simulink model "Concave_hipp"  (R2023a)
settings: Solver=ode3  StartTime=0.0  StopTime=100  FixedStep=0.0001  RelTol=1e-3
values from neighbouring files (symbols this model uses):
  d_pitch_2 = 1    [simulation_para.m]
  d_roll_2 = 1    [simulation_para.m]
  d_yaw_2 = 1    [simulation_para.m]
  disturbance = 0    [simulation_para.m]
  dpitch_para = [1,1,1,0.01]    [simulation_para.m]
  droll_para = [1,1,1,0.01]    [simulation_para.m]
  dyaw_para = [1,1,1,0.01]    [simulation_para.m]
  k_pos_2 = 8    [simulation_para.m]
  k_vel_2 = 8    [simulation_para.m]
  kp_para = [8,20,1,0.01]    [simulation_para.m]
  kv_para = [8,20,1,0.01]    [simulation_para.m]
  p_pitch_2 = 10    [simulation_para.m]
  p_roll_2 = 10    [simulation_para.m]
  p_yaw_2 = 10    [simulation_para.m]
  ppitch_para = [10,10,1,0.01]    [simulation_para.m]
  proll_para = [10,10,1,0.01]    [simulation_para.m]
  pyaw_para = [10,20,1,0.01]    [simulation_para.m]
  Q1 = -8    [simulation_para.m]
  Q2 = -10    [simulation_para.m]
  Q3 = -[0.01,5,8]    [simulation_para.m]
  Q4 = -[0.001,0.1,0.1]    [simulation_para.m]
  Qc1 = -[8,50,1,0.01]    [simulation_para.m]
  Qc2 = -[10,80,1,0.02]    [simulation_para.m]
  Qc3 = [qc3_1;qc3_2;qc3_3]    [simulation_para.m]
  Qc4 = [qc4_1;qc4_2;qc4_3]    [simulation_para.m]
(part 1 of 2)
settings Model: Creator=fansh  LastModifiedBy=fansh
settings DebuggingCC: MultiTaskCondExecSysMsg=none  MultiTaskRateTransMsg=warning  TasksWithSamePriorityMsg=none  SigSpecEnsureSampleTimeMsg=none  UnknownTsInhSupMsg=none  SFUnexpectedBacktrackingDiag=none

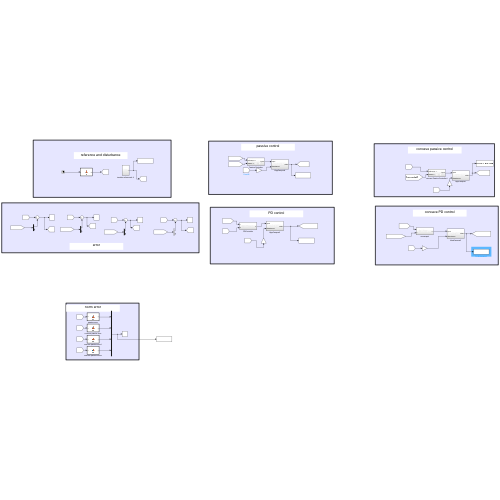
[thumbnail: Simulink's stored preview of the top-level diagram]
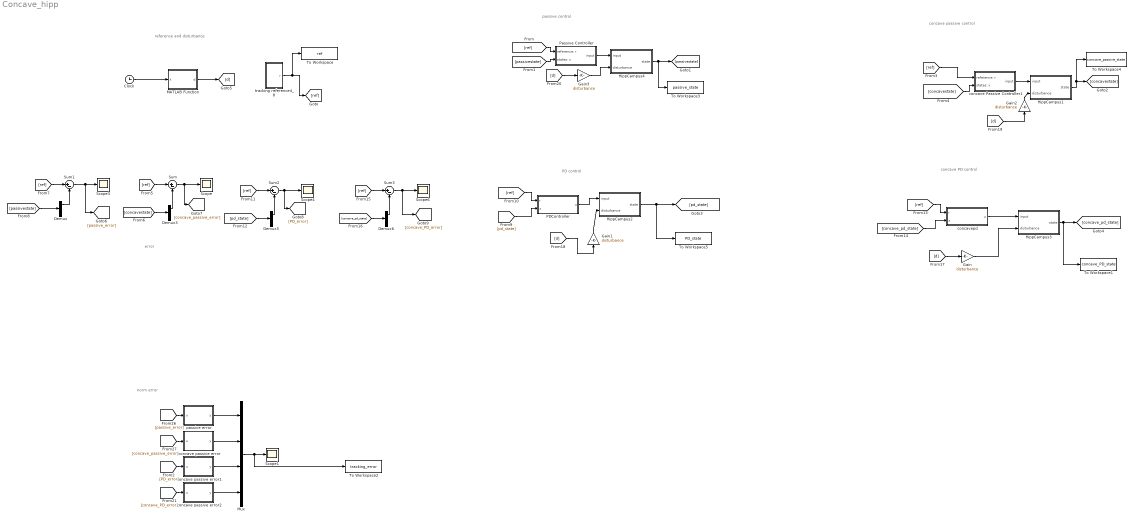
== system Concave_hipp ==
  note: concave passive control
  note: passive control
  note: PD control
  note: concave PD control
  note: reference and disturbance
  note: error
  note: norm error
  Clock : Clock
  Demux{,3,5..6} (4 alike) : Demux  Outputs=[3 9]
  Gain{,1..3} (4 alike) : Gain  Gain=disturbance
  HippCampus1 : Subsystem
  HippCampus2 : Subsystem
  HippCampus3 : Subsystem
  HippCampus4 : Subsystem
  MATLAB Function : MATLAB Function  TreatAsAtomicUnit=on
  Mux : Mux
  PDController : Subsystem
  Passive Controller : Subsystem
  Scope{,1,3..4,6} (5 alike) : Scope
  Sum{,1..3} (4 alike) : Sum  Inputs=|+-
  To Workspace : ToWorkspace  VariableName=ref  SaveFormat=Timeseries  SampleTime=-1
  To Workspace1 : ToWorkspace  VariableName=concave_PD_state  SaveFormat=Timeseries  SampleTime=-1
  To Workspace2 : ToWorkspace  VariableName=tracking_error  SaveFormat=Timeseries  SampleTime=-1
  To Workspace3 : ToWorkspace  VariableName=passive_state  SaveFormat=Timeseries  SampleTime=-1
  To Workspace4 : ToWorkspace  VariableName=concave_passive_state  SaveFormat=Timeseries  SampleTime=-1
  To Workspace5 : ToWorkspace  VariableName=PD_state  SaveFormat=Timeseries  SampleTime=-1
  concave Passive Controller1 : Subsystem
  concave passive error : MATLAB Function  TreatAsAtomicUnit=on
  concave passive error1 : MATLAB Function  TreatAsAtomicUnit=on
  concave passive error2 : MATLAB Function  TreatAsAtomicUnit=on
  concavepd : Subsystem
  passive error : MATLAB Function  TreatAsAtomicUnit=on
  tracking reference4_8 : Subsystem
  wires:
  Passive Controller/1(input) -> HippCampus4/1(input)
  HippCampus4/1(state) -> To Workspace3/1, [passivestate]
  [ref] -> Passive Controller/1(reference: r)
  [passivestate] -> Passive Controller/2(states: x)
  [ref] -> concave Passive Controller1/1(reference: r)
  concave Passive Controller1/1(input) -> HippCampus1/1(input)
  [concavestate] -> concave Passive Controller1/2(states: x)
  HippCampus1/1(state) -> To Workspace4/1, [concavestate]
  [ref] -> Sum/1
  [concavestate] -> Demux3/1
  Sum/1 -> [concave_passive_error], Scope/1
  [passivestate] -> Demux/1
  Sum1/1 -> [passive_error], Scope3/1
  [ref] -> Sum1/1
  Demux/1 -> Sum1/2
  Demux3/1 -> Sum/2
  PDController/1(u) -> HippCampus2/1(input)
  [ref] -> PDController/1(r)
  HippCampus2/1(state) -> To Workspace5/1, [pd_state]
  [pd_state] -> PDController/2(x)
  Sum2/1 -> [PD_error], Scope4/1
  [ref] -> Sum2/1
  [pd_state] -> Demux5/1
  Demux5/1 -> Sum2/2
  [ref] -> concavepd/1(r)
  HippCampus3/1(state) -> To Workspace1/1, [concave_pd_state]
  [concave_pd_state] -> concavepd/2(x)
  concavepd/1(u) -> HippCampus3/1(input)
  [concave_pd_state] -> Demux6/1
  [ref] -> Sum3/1
  Demux6/1 -> Sum3/2
  Sum3/1 -> [concave_PD_error], Scope6/1
  Clock/1 -> MATLAB Function/1(t)
  MATLAB Function/1(d) -> [d]
  [d] -> Gain/1
  tracking reference4_8/1(r) -> [ref], To Workspace/1
  Gain/1 -> HippCampus3/2(disturbance)
  [d] -> Gain1/1
  [d] -> Gain2/1
  [d] -> Gain3/1
  Gain1/1 -> HippCampus2/2(disturbance)
  Gain2/1 -> HippCampus1/2(disturbance)
  Gain3/1 -> HippCampus4/2(disturbance)
  [passive_error] -> passive error/1(u)
  [concave_passive_error] -> concave passive error/1(u)
  [PD_error] -> concave passive error1/1(u)
  [concave_PD_error] -> concave passive error2/1(u)
  passive error/1(y) -> Mux/1
  concave passive error/1(y) -> Mux/2
  concave passive error1/1(y) -> Mux/3
  concave passive error2/1(y) -> Mux/4
  Mux/1 -> To Workspace2/1, Scope1/1

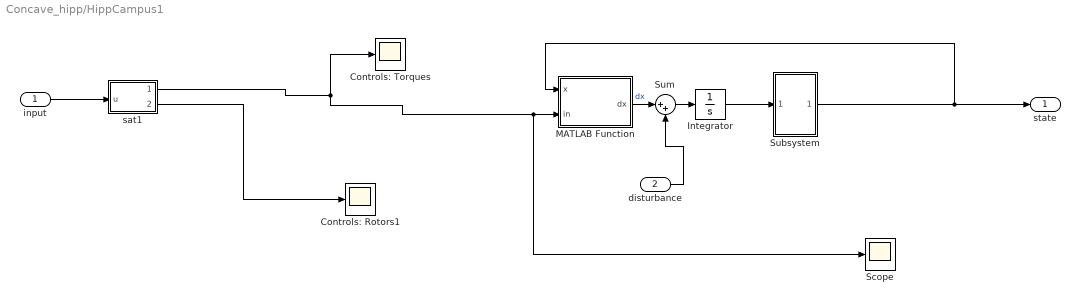
== system Concave_hipp/HippCampus1 ==
  input : Inport
  disturbance : Inport  Port=2
  Controls: Rotors1 : Scope
  Controls: Torques : Scope
  Integrator : Integrator  InitialCondition=zeros(12,1)
  MATLAB Function : MATLAB Function  TreatAsAtomicUnit=on
  Scope : Scope
  Subsystem : Subsystem
  Sum : Sum  Inputs=|++
  sat1 : MATLAB Function  TreatAsAtomicUnit=on
  state : Outport
  wires:
  MATLAB Function/1(dx) -> Sum/1  "dx"
  Integrator/1 -> Subsystem/1(In1)
  sat1/1(u_sat) -> Controls: Torques/1, MATLAB Function/2(in), Scope/1
  Subsystem/1(state) -> MATLAB Function/1(x), state/1
  input/1 -> sat1/1(u)
  sat1/2(omega) -> Controls: Rotors1/1
  Sum/1 -> Integrator/1
  disturbance/1 -> Sum/2

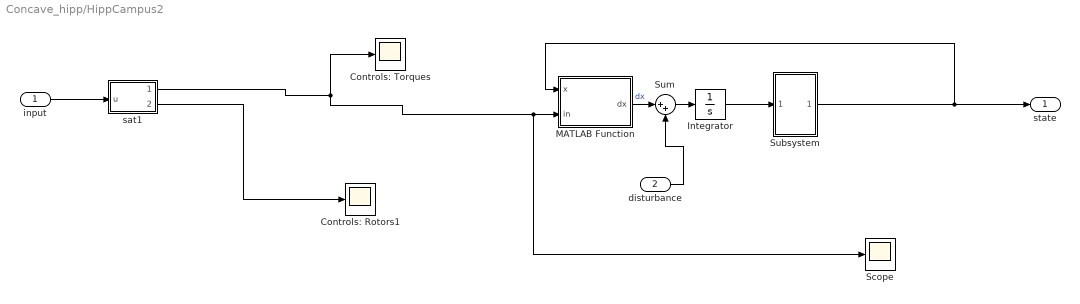
== system Concave_hipp/HippCampus2 ==
  input : Inport
  disturbance : Inport  Port=2
  Controls: Rotors1 : Scope
  Controls: Torques : Scope
  Integrator : Integrator  InitialCondition=zeros(12,1)
  MATLAB Function : MATLAB Function  TreatAsAtomicUnit=on
  Scope : Scope
  Subsystem : Subsystem
  Sum : Sum  Inputs=|++
  sat1 : MATLAB Function  TreatAsAtomicUnit=on
  state : Outport
  wires:
  MATLAB Function/1(dx) -> Sum/1  "dx"
  Integrator/1 -> Subsystem/1(In1)
  sat1/1(u_sat) -> Controls: Torques/1, MATLAB Function/2(in), Scope/1
  Subsystem/1(state) -> MATLAB Function/1(x), state/1
  input/1 -> sat1/1(u)
  sat1/2(omega) -> Controls: Rotors1/1
  Sum/1 -> Integrator/1
  disturbance/1 -> Sum/2

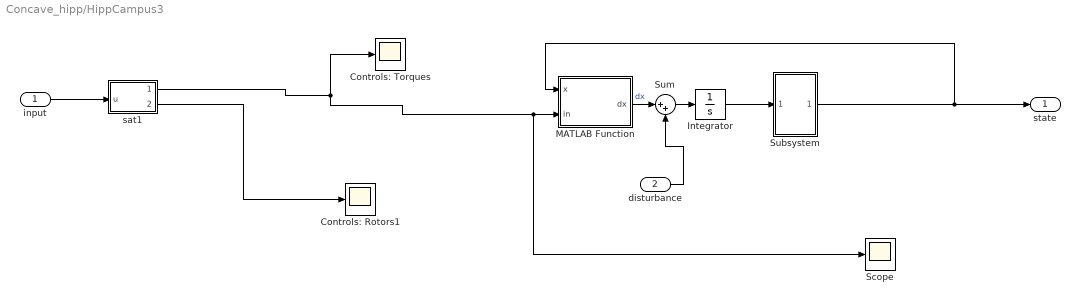
== system Concave_hipp/HippCampus3 ==
  input : Inport
  disturbance : Inport  Port=2
  Controls: Rotors1 : Scope
  Controls: Torques : Scope
  Integrator : Integrator  InitialCondition=zeros(12,1)
  MATLAB Function : MATLAB Function  TreatAsAtomicUnit=on
  Scope : Scope
  Subsystem : Subsystem
  Sum : Sum  Inputs=|++
  sat1 : MATLAB Function  TreatAsAtomicUnit=on
  state : Outport
  wires:
  MATLAB Function/1(dx) -> Sum/1  "dx"
  Integrator/1 -> Subsystem/1(In1)
  sat1/1(u_sat) -> Controls: Torques/1, MATLAB Function/2(in), Scope/1
  Subsystem/1(state) -> MATLAB Function/1(x), state/1
  input/1 -> sat1/1(u)
  sat1/2(omega) -> Controls: Rotors1/1
  Sum/1 -> Integrator/1
  disturbance/1 -> Sum/2

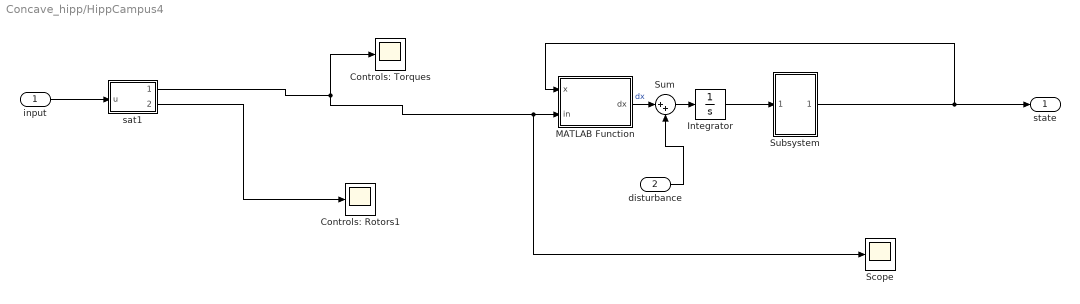
== system Concave_hipp/HippCampus4 ==
  input : Inport
  disturbance : Inport  Port=2
  Controls: Rotors1 : Scope
  Controls: Torques : Scope
  Integrator : Integrator  InitialCondition=zeros(12,1)
  MATLAB Function : MATLAB Function  TreatAsAtomicUnit=on
  Scope : Scope
  Subsystem : Subsystem
  Sum : Sum  Inputs=|++
  sat1 : MATLAB Function  TreatAsAtomicUnit=on
  state : Outport
  wires:
  MATLAB Function/1(dx) -> Sum/1  "dx"
  Integrator/1 -> Subsystem/1(In1)
  sat1/1(u_sat) -> Controls: Torques/1, MATLAB Function/2(in), Scope/1
  Subsystem/1(state) -> MATLAB Function/1(x), state/1
  input/1 -> sat1/1(u)
  sat1/2(omega) -> Controls: Rotors1/1
  Sum/1 -> Integrator/1
  disturbance/1 -> Sum/2

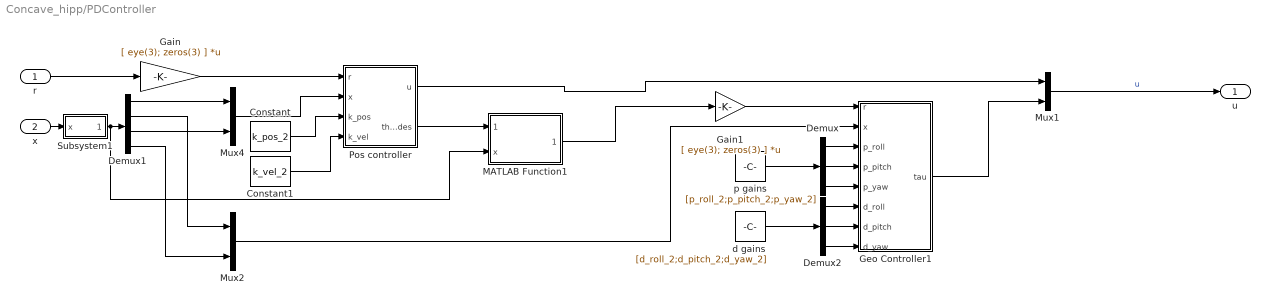
== system Concave_hipp/PDController ==
  r : Inport
  x : Inport  Port=2
  Constant : Constant  Value=k_pos_2
  Constant1 : Constant  Value=k_vel_2
  Demux : Demux  Outputs=3
  Demux1 : Demux  Outputs=[3 3 3 3]
  Demux2 : Demux  Outputs=3
  Gain : Gain  Gain=[ eye(3); zeros(3) ]  Multiplication=Matrix(K*u) (u vector)
  Gain1 : Gain  Gain=[ eye(3); zeros(3) ]  Multiplication=Matrix(K*u) (u vector)
  Geo Controller1 : MATLAB Function  TreatAsAtomicUnit=on
  MATLAB Function1 : MATLAB Function  TreatAsAtomicUnit=on
  Mux1 : Mux  Inputs=2
  Mux2 : Mux  Inputs=2
  Mux4 : Mux  Inputs=2
  Pos controller : MATLAB Function  TreatAsAtomicUnit=on
  Subsystem1 : Subsystem
  d gains : Constant  Value=[d_roll_2;d_pitch_2;d_yaw_2]
  p gains : Constant  Value=[p_roll_2;p_pitch_2;p_yaw_2]
  u : Outport
  wires:
  Geo Controller1/1(tau) -> Mux1/2
  Mux1/1 -> u/1  "u"
  Pos controller/1(u) -> Mux1/1
  x/1 -> Subsystem1/1(x)
  Demux1/1 -> Mux4/1
  Demux1/3 -> Mux4/2
  Mux4/1 -> Pos controller/2(x)
  Demux1/2 -> Mux2/1
  Demux1/4 -> Mux2/2
  Mux2/1 -> Geo Controller1/2(x)
  Pos controller/2(theta_des) -> MATLAB Function1/1("theta_des ")
  Gain1/1 -> Geo Controller1/1(r)
  r/1 -> Gain/1
  Gain/1 -> Pos controller/1(r)
  Constant/1 -> Pos controller/3(k_pos)
  Constant1/1 -> Pos controller/4(k_vel)
  Demux/3 -> Geo Controller1/5(p_yaw)
  Demux/2 -> Geo Controller1/4(p_pitch)
  p gains/1 -> Demux/1
  Demux2/3 -> Geo Controller1/8(d_yaw)
  Demux2/2 -> Geo Controller1/7(d_pitch)
  Demux/1 -> Geo Controller1/3(p_roll)
  Demux2/1 -> Geo Controller1/6(d_roll)
  d gains/1 -> Demux2/1
  MATLAB Function1/1(theta_des) -> Gain1/1
  Subsystem1/1(x_2pi) -> MATLAB Function1/2(x), Demux1/1

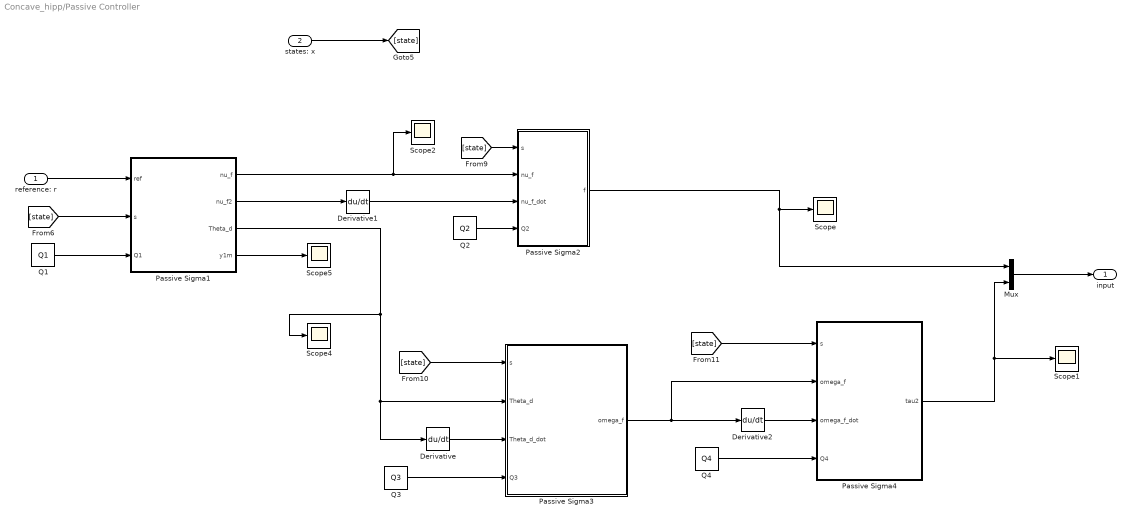
== system Concave_hipp/Passive Controller ==
  reference: r : Inport
  states: x : Inport  Port=2
  Derivative : Derivative
  Derivative1 : Derivative
  Derivative2 : Derivative
  Mux : Mux  Inputs=2
  Passive Sigma1 : MATLAB Function  TreatAsAtomicUnit=on
  Passive Sigma2 : MATLAB Function  TreatAsAtomicUnit=on
  Passive Sigma3 : MATLAB Function  TreatAsAtomicUnit=on
  Passive Sigma4 : MATLAB Function  TreatAsAtomicUnit=on
  Q1 : Constant  Value=Q1
  Q2 : Constant  Value=Q2
  Q3 : Constant  Value=Q3
  Q4 : Constant  Value=Q4
  Scope{,1..2,4..5} (5 alike) : Scope
  input : Outport
  wires:
  reference: r/1 -> Passive Sigma1/1(ref)
  states: x/1 -> [state]
  Q1/1 -> Passive Sigma1/3(Q1)
  [state] -> Passive Sigma1/2(s)
  Passive Sigma1/1(nu_f) -> Passive Sigma2/2(nu_f), Scope2/1
  [state] -> Passive Sigma2/1(s)
  [state] -> Passive Sigma3/1(s)
  [state] -> Passive Sigma4/1(s)
  Q2/1 -> Passive Sigma2/4(Q2)
  Q3/1 -> Passive Sigma3/4(Q3)
  Q4/1 -> Passive Sigma4/4(Q4)
  Mux/1 -> input/1
  Passive Sigma1/2(nu_f2) -> Derivative1/1
  Derivative/1 -> Passive Sigma3/3(Theta_d_dot)
  Derivative2/1 -> Passive Sigma4/3(omega_f_dot)
  Passive Sigma2/1(f) -> Mux/1, Scope/1
  Passive Sigma4/1(tau2) -> Mux/2, Scope1/1
  Passive Sigma1/4(y1m) -> Scope5/1
  Derivative1/1 -> Passive Sigma2/3(nu_f_dot)
  Passive Sigma1/3(Theta_d) -> Passive Sigma3/2(Theta_d), Derivative/1, Scope4/1
  Passive Sigma3/1(omega_f) -> Passive Sigma4/2(omega_f), Derivative2/1

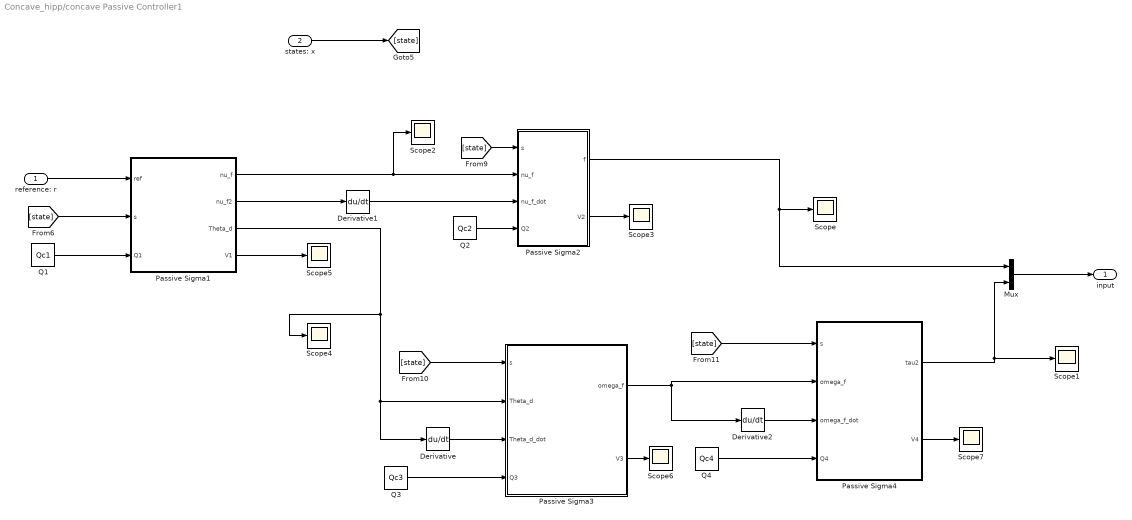
== system Concave_hipp/concave Passive Controller1 ==
  reference: r : Inport
  states: x : Inport  Port=2
  Derivative : Derivative
  Derivative1 : Derivative
  Derivative2 : Derivative
  Mux : Mux  Inputs=2
  Passive Sigma1 : MATLAB Function  TreatAsAtomicUnit=on
  Passive Sigma2 : MATLAB Function  TreatAsAtomicUnit=on
  Passive Sigma3 : MATLAB Function  TreatAsAtomicUnit=on
  Passive Sigma4 : MATLAB Function  TreatAsAtomicUnit=on
  Q1 : Constant  Value=Qc1
  Q2 : Constant  Value=Qc2
  Q3 : Constant  Value=Qc3
  Q4 : Constant  Value=Qc4
  Scope{,1..7} (8 alike) : Scope
  input : Outport
  wires:
  reference: r/1 -> Passive Sigma1/1(ref)
  states: x/1 -> [state]
  Q1/1 -> Passive Sigma1/3(Q1)
  [state] -> Passive Sigma1/2(s)
  Passive Sigma1/1(nu_f) -> Passive Sigma2/2(nu_f), Scope2/1
  [state] -> Passive Sigma2/1(s)
  [state] -> Passive Sigma3/1(s)
  [state] -> Passive Sigma4/1(s)
  Q2/1 -> Passive Sigma2/4(Q2)
  Q3/1 -> Passive Sigma3/4(Q3)
  Q4/1 -> Passive Sigma4/4(Q4)
  Mux/1 -> input/1
  Passive Sigma1/2(nu_f2) -> Derivative1/1
  Derivative/1 -> Passive Sigma3/3(Theta_d_dot)
  Derivative2/1 -> Passive Sigma4/3(omega_f_dot)
  Passive Sigma2/1(f) -> Mux/1, Scope/1
  Passive Sigma4/1(tau2) -> Mux/2, Scope1/1
  Passive Sigma1/4(V1) -> Scope5/1
  Derivative1/1 -> Passive Sigma2/3(nu_f_dot)
  Passive Sigma1/3(Theta_d) -> Passive Sigma3/2(Theta_d), Derivative/1, Scope4/1
  Passive Sigma3/1(omega_f) -> Derivative2/1, Passive Sigma4/2(omega_f)
  Passive Sigma2/2(V2) -> Scope3/1
  Passive Sigma3/2(V3) -> Scope6/1
  Passive Sigma4/2(V4) -> Scope7/1

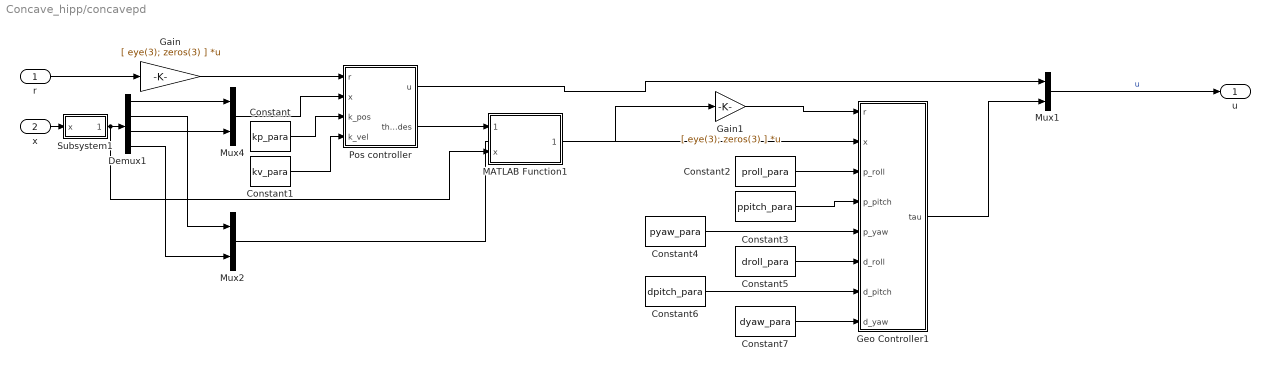
== system Concave_hipp/concavepd ==
  r : Inport
  x : Inport  Port=2
  Constant : Constant  Value=kp_para
  Constant1 : Constant  Value=kv_para
  Constant2 : Constant  Value=proll_para
  Constant3 : Constant  Value=ppitch_para
  Constant4 : Constant  Value=pyaw_para
  Constant5 : Constant  Value=droll_para
  Constant6 : Constant  Value=dpitch_para
  Constant7 : Constant  Value=dyaw_para
  Demux1 : Demux  Outputs=[3 3 3 3]
  Gain : Gain  Gain=[ eye(3); zeros(3) ]  Multiplication=Matrix(K*u) (u vector)
  Gain1 : Gain  Gain=[ eye(3); zeros(3) ]  Multiplication=Matrix(K*u) (u vector)
  Geo Controller1 : MATLAB Function  TreatAsAtomicUnit=on
  MATLAB Function1 : MATLAB Function  TreatAsAtomicUnit=on
  Mux1 : Mux  Inputs=2
  Mux2 : Mux  Inputs=2
  Mux4 : Mux  Inputs=2
  Pos controller : MATLAB Function  TreatAsAtomicUnit=on
  Subsystem1 : Subsystem
  u : Outport
  wires:
  Geo Controller1/1(tau) -> Mux1/2
  Mux1/1 -> u/1  "u"
  Pos controller/1(u) -> Mux1/1
  x/1 -> Subsystem1/1(x)
  Demux1/1 -> Mux4/1
  Demux1/3 -> Mux4/2
  Mux4/1 -> Pos controller/2(x)
  Demux1/2 -> Mux2/1
  Demux1/4 -> Mux2/2
  Mux2/1 -> Geo Controller1/2(x)
  Pos controller/2(theta_des) -> MATLAB Function1/1("theta_des ")
  Gain1/1 -> Geo Controller1/1(r)
  r/1 -> Gain/1
  Gain/1 -> Pos controller/1(r)
  Constant/1 -> Pos controller/3(k_pos)
  Constant1/1 -> Pos controller/4(k_vel)
  Constant2/1 -> Geo Controller1/3(p_roll)
  MATLAB Function1/1(theta_des) -> Gain1/1
  Subsystem1/1(x_2pi) -> MATLAB Function1/2(x), Demux1/1
  Constant3/1 -> Geo Controller1/4(p_pitch)
  Constant4/1 -> Geo Controller1/5(p_yaw)
  Constant5/1 -> Geo Controller1/6(d_roll)
  Constant6/1 -> Geo Controller1/7(d_pitch)
  Constant7/1 -> Geo Controller1/8(d_yaw)

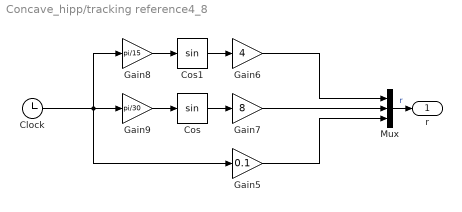
== system Concave_hipp/tracking reference4_8 ==
  Clock : Clock
  Cos : Trigonometry
  Cos1 : Trigonometry
  Gain5 : Gain  Gain=0.1
  Gain6 : Gain  Gain=4
  Gain7 : Gain  Gain=8
  Gain8 : Gain  Gain=pi/15
  Gain9 : Gain  Gain=pi/30
  Mux : Mux  Inputs=3
  r : Outport
  wires:
  Gain9/1 -> Cos/1
  Gain6/1 -> Mux/1
  Gain7/1 -> Mux/2
  Cos1/1 -> Gain6/1
  Cos/1 -> Gain7/1
  Mux/1 -> r/1  "r"
  Gain8/1 -> Cos1/1
  Gain5/1 -> Mux/3
  Clock/1 -> Gain5/1, Gain9/1, Gain8/1

== system Concave_hipp/HippCampus1/Subsystem ==
  In1 : Inport
  Demux : Demux  Outputs=[5 1 1 1 4]
  Mux : Mux  Inputs=5
  state : Outport
  wires:
  Demux/2 -> Mux/2
  In1/1 -> Demux/1
  Demux/3 -> Mux/3
  Demux/1 -> Mux/1
  Mux/1 -> state/1
  Demux/5 -> Mux/5
  Demux/4 -> Mux/4

== system Concave_hipp/HippCampus2/Subsystem ==
  In1 : Inport
  Demux : Demux  Outputs=[5 1 1 1 4]
  Mux : Mux  Inputs=5
  state : Outport
  wires:
  Demux/2 -> Mux/2
  In1/1 -> Demux/1
  Demux/3 -> Mux/3
  Demux/1 -> Mux/1
  Mux/1 -> state/1
  Demux/5 -> Mux/5
  Demux/4 -> Mux/4

== system Concave_hipp/HippCampus3/Subsystem ==
  In1 : Inport
  Demux : Demux  Outputs=[5 1 1 1 4]
  Mux : Mux  Inputs=5
  state : Outport
  wires:
  Demux/2 -> Mux/2
  In1/1 -> Demux/1
  Demux/3 -> Mux/3
  Demux/1 -> Mux/1
  Mux/1 -> state/1
  Demux/5 -> Mux/5
  Demux/4 -> Mux/4

== system Concave_hipp/HippCampus4/Subsystem ==
  In1 : Inport
  Demux : Demux  Outputs=[5 1 1 1 4]
  Mux : Mux  Inputs=5
  state : Outport
  wires:
  Demux/2 -> Mux/2
  In1/1 -> Demux/1
  Demux/3 -> Mux/3
  Demux/1 -> Mux/1
  Mux/1 -> state/1
  Demux/5 -> Mux/5
  Demux/4 -> Mux/4

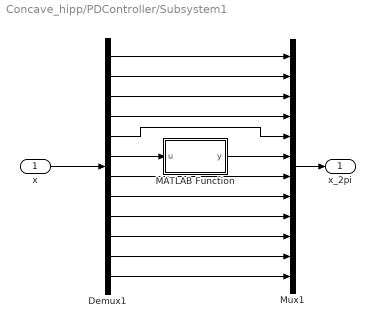
== system Concave_hipp/PDController/Subsystem1 ==
  x : Inport
  Demux1 : Demux  Outputs=12
  MATLAB Function : MATLAB Function  TreatAsAtomicUnit=on
  Mux1 : Mux  Inputs=12
  x_2pi : Outport
  wires:
  Mux1/1 -> x_2pi/1
  x/1 -> Demux1/1
  Demux1/6 -> MATLAB Function/1(u)
  Demux1/1 -> Mux1/1
  Demux1/2 -> Mux1/2
  Demux1/3 -> Mux1/3
  Demux1/4 -> Mux1/4
  Demux1/5 -> Mux1/5
  Demux1/7 -> Mux1/7
  Demux1/8 -> Mux1/8
  Demux1/9 -> Mux1/9
  Demux1/10 -> Mux1/10
  Demux1/11 -> Mux1/11
  Demux1/12 -> Mux1/12
  MATLAB Function/1(y) -> Mux1/6

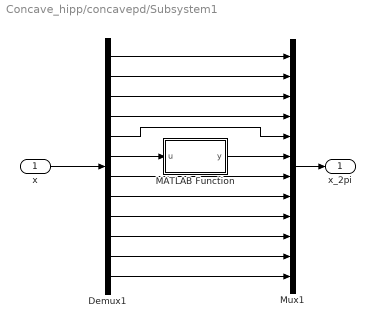
== system Concave_hipp/concavepd/Subsystem1 ==
  x : Inport
  Demux1 : Demux  Outputs=12
  MATLAB Function : MATLAB Function  TreatAsAtomicUnit=on
  Mux1 : Mux  Inputs=12
  x_2pi : Outport
  wires:
  Mux1/1 -> x_2pi/1
  x/1 -> Demux1/1
  Demux1/6 -> MATLAB Function/1(u)
  Demux1/1 -> Mux1/1
  Demux1/2 -> Mux1/2
  Demux1/3 -> Mux1/3
  Demux1/4 -> Mux1/4
  Demux1/5 -> Mux1/5
  Demux1/7 -> Mux1/7
  Demux1/8 -> Mux1/8
  Demux1/9 -> Mux1/9
  Demux1/10 -> Mux1/10
  Demux1/11 -> Mux1/11
  Demux1/12 -> Mux1/12
  MATLAB Function/1(y) -> Mux1/6

== matlab function Concave_hipp/HippCampus4/sat1 ==
  data: u input; u_sat output; omega output
function [u_sat, omega] = fcn(u)
  %  u_sat=u;
    h     = 0.0481;   % [m] Distance of rotors to HippoCampus center
    Cd    = 0.0024;   % Coefficient of drag for the rotors
    tlim  = 3;        % Maximal torque of the motors 

    Q = [1,1,1,1;-Cd,Cd,-Cd,Cd;-h,-h,h,h;h,-h,-h,h];
    Qinv = inv(Q);

    % Transform into rotor space
    omega = Qinv*u;

    % Calculate utilization of each rotor
    util  = abs(omega/tlim);

    % Saturate torque at max utilization
    omega = omega ./ max(util, 1);    

    %Transform back into body frame
   u_sat = Q * omega;
end

== matlab function Concave_hipp/HippCampus2/MATLAB Function ==
  data: x input; dx output; in input

function dx = fcn(x, in)
zg    =  0.05;    % [m]
g     =  9.81;    % [m/s^2]

m     =  1.43;    % [kg]
Ix    = 0.00241; % [kgm^2]
Iy    = 0.01072; % [kgm^2]
Iz    = 0.01072; % [kgm^2]
Xudot = -1.11;    % [kg]
Yvdot = -2.80;    % [kg]
Zwdot = -2.80;    % [kg]
Kpdot = -0.0018;  % [kgm^2]
Mqdot = -0.0095;  % [kgm^2]
Nrdot = -0.0095;  % [kgm^2]
Xu    = -4.56;    % [kg/m]
Yv    = -17.36;   % [kg/m]
Zw    = -17.36;   % [kg/m]
Kp    = -0.0028;  % [kgm^2]
Mq    = -0.0476;  % [kgm^2]
Nr    = -0.0476;  % [kgm^2]
% Extract states into more readable form
phi = x( 4); theta = x( 5);
u   = x( 7); v     = x( 8); w   = x( 9);
p   = x(10); q     = x(11); r   = x(12);
nu  = x(7:12);

% Construct rotational tensor
R = body_frame_rotation(x(4:6));

% Construct velocity transformation tensor
T = [ 1  sin(phi)*tan(theta)   cos(phi)*tan(theta) ;
    0  cos(phi)             -sin(phi)            ;
    0  sin(phi)/cos(theta)   cos(phi)/cos(theta) ];
J = [ R         zeros(3) ;
    zeros(3)  T        ];

% Calculate mass matrix
Ma  = -diag([Xudot, Yvdot, Zwdot, Kpdot, Mqdot, Nrdot]);
Mrb =  diag([m,  m,  m, Ix, Iy, Iz]);
M = Ma + Mrb;

% Compute hydrostatic load
gravity = zg * g * m;
G = [ 0; 0; 0; gravity * cos(theta) * sin(phi); gravity * sin(theta); 0 ];

% Construct coriolis matrix, see Fossen 2011, Theorem 3.2
C12 = -skew(M(1:3,1:3) * nu(1:3));
C = [ zeros(3)   C12                        ;
    C12       -skew(M(4:6,4:6) * nu(4:6)) ];

% Construct damping matrix
D = -diag([Xu * abs(u), Yv * abs(v),...
    Zw * abs(w), Kp * abs(p),...
    Mq * abs(q), Nr * abs(r)]);

% Build state space equations
tau  = [ in(1); 0; 0; in(2:4) ];

dx       = zeros(12,1);
dx(1:6)  = J*nu;
dx(7:12) = M \ (tau - (C+D)*nu - G);
end

== matlab function Concave_hipp/HippCampus2/sat1 ==
  data: u input; u_sat output; omega output
function [u_sat, omega] = fcn(u)
  %  u_sat=u;
    h     = 0.0481;   % [m] Distance of rotors to HippoCampus center
    Cd    = 0.0024;   % Coefficient of drag for the rotors
    tlim  = 3;        % Maximal torque of the motors 

    Q = [1,1,1,1;-Cd,Cd,-Cd,Cd;-h,-h,h,h;h,-h,-h,h];
    Qinv = inv(Q);

    % Transform into rotor space
    omega = Qinv*u;

    % Calculate utilization of each rotor
    util  = abs(omega/tlim);

    % Saturate torque at max utilization
    omega = omega ./ max(util, 1);    

    %Transform back into body frame
   u_sat = Q * omega;
end

== matlab function Concave_hipp/PDController/Pos controller ==
  data: r input; x input; u output; theta_des output; k_pos input; k_vel input
function [u,theta_des] = fcn(r, x,k_pos,k_vel)
%% Heuristic position controller
% Just wrap around a hueristic position controller around the attitude
% controller
%
% Gains that work for backup
% k_pos=2;
% k_vel=2;

drive_forward=1; % Easier to drive the unicycle backward than forward
if drive_forward==1
    e=r(1:3,1)-x(1:3,1);
    v_des=k_pos*norm(e,2);
else
    e=x(1:3,1)-r(1:3,1);
    v_des=-k_pos*norm(e,2);    
end
u=k_vel*(v_des-x(4));
proj_dist_xy=norm(e(1:2,1),2);
pitch_des=-atan2(e(3,1),proj_dist_xy);
psi_des=atan2(e(2),e(1));
theta_des=[0;pitch_des;psi_des]; 
end

== matlab function Concave_hipp/concave Passive Controller1/Passive Sigma1 ==
  data: ref input; nu_f output; nu_f2 output; s input; Q1 input; Theta_d output; V1 output
%---------------------------------------------------------------------------------------------
% For Paper, 
% "Three-Dimensional Simultaneous Stabilization and Tracking Control of Nonholonomic Autonomous Underwater Vehicles"
% by Shuyuan Fan and Herbert Werner
% Copyright (c) Institute of Control Systems, Hamburg University of Technology. All rights reserved.
% Licensed under the GPLv3. See LICENSE in the project root for license information.
% Uses an own implementation of the work of 
% IEEE Conference on Decision and Control and L-CSS, 2022."
% Author(s): Shuyuan Fan
%--------------------------------------------------------------------------------------------
function [nu_f,nu_f2,Theta_d,V1]= fcn(ref,s,Q1)
zg    =  0.05;    % [m]
g     =  9.81;    % [m/s^2]

m     =  1.43;    % [kg]
Ix    = 0.00241; % [kgm^2]
Iy    = 0.01072; % [kgm^2]
Iz    = 0.01072; % [kgm^2]
Xudot = -1.11;    % [kg]
Yvdot = -2.80;    % [kg]
Zwdot = -2.80;    % [kg]
Kpdot = -0.0018;  % [kgm^2]
Mqdot = -0.0095;  % [kgm^2]
Nrdot = -0.0095;  % [kgm^2]
Xu    = -4.56;    % [kg/m]
Yv    = -17.36;   % [kg/m]
Zw    = -17.36;   % [kg/m]
Kp    = -0.0028;  % [kgm^2]
Mq    = -0.0476;  % [kgm^2]
Nr    = -0.0476;  % [kgm^2]

% Calculate mass matrix
Ma  = -diag([Xudot, Yvdot, Zwdot, Kpdot, Mqdot, Nrdot]);
Mrb =  diag([m,  m,  m, Ix, Iy, Iz]);
M = Ma + Mrb;

M1 = M(1:3,1:3);
%% reference
x_ref = ref(1);
y_ref = ref(2);
z_ref = ref(3);
Xref = [x_ref;y_ref;z_ref];

%% states
x = s(1); y = s(2); z = s(3);
X = s(1:3);

angle = s(4:6);
phi = s(4);
%phi =min(max(phi,-0.5),0.5);
theta = s(5); 
%theta = min(max(theta,-1.5),1.5);
psi = s(6);
%psi =  wrapToPi(psi);
nu = s(7:9) ;
u=s(7); v=s(8); w=s(9); 

omega = s(10:12);
p=s(10); q=s(11); r=s(12);

% storage function V1
V1 = 0.5*(X-Xref)'*(X-Xref);

% Gamma function for nu
if u<0.5
    nu_u = 0.5;
else
    nu_u = u;
end

nu = [nu_u;v;w];
Gamma_nu = vectortodirect(nu);


% R(Theta)
Rotation = body_frame_rotation(angle);
y1m = Gamma_nu'*Rotation'*(X-Xref);

Q1 = -sliderconcave(V1,-Q1);
nu_f = Q1*y1m;
nu_f2 = Gamma_nu*nu_f;

%% Theta_d

Xe = X-Xref;
phi_d  = 0;
theta_d = atan2(Xe(3),sqrt(Xe(1)^2+Xe(2)^2)+eps);
psi_d = atan2(-Xe(2),-Xe(1));
psi_d = wrapTo2Pi(psi_d);
Theta_d = [phi_d;theta_d;psi_d];
end

== matlab function Concave_hipp/PDController/Subsystem1/MATLAB Function ==
  data: u input; y output
function y = fcn(u)
y = mod(u + pi, 2*pi) - pi;

== matlab function Concave_hipp/concavepd/Geo Controller1 ==
  data: r input; x input; tau output; p_roll input; p_pitch input; p_yaw input; d_roll input; d_pitch input; d_yaw input
function tau = fcn(r, x,p_roll,p_pitch,p_yaw,d_roll,d_pitch,d_yaw)
%% Geo Controller following
% D. Mellinger and V. Kumar. Minimum Snap Trajectory Generation and Control
% for Quadrotors. ICRA, 2011
% D.A. Duecker,  A. Hackbarth, T. Johannink, E. Kreuzer, and E. Solowjow. 
% Micro Underwater Vehicle Hydrobatics: A Submerged Furuta Pendulum. ICRA,
% 2018.
%

% Gains that work for backup
% p_roll  = 4;
% p_pitch = 4;
% p_yaw   = 4;
% 
% d_roll  = 1.5;
% d_pitch = 2;
% d_yaw   = 2;


%% Transform attitude into SO(3)
Phi     = x(1:3);
Phi_des = r(1:3);

R       = R_euler(Phi);
R_des   = R_euler(Phi_des);

%% Compute control errors

% Compute attitude error on SO(3)
e_R = 0.5*(R_des'*R - R'*R_des);

% Extract the skew-symmetric part of the rotation error matrix as a vector
e_R_vec = [e_R(3,2); e_R(1,3); e_R(2,1)]; 

p_roll = sliderconcave(e_R(3,2)*2,p_roll);
p_pitch = sliderconcave(e_R(1,3)*2,p_pitch);
p_yaw = sliderconcave(e_R(2,1)*2,p_yaw);
K_p = diag([p_roll, p_pitch, p_yaw]);



% Compute the error in the angular velocities
omega     = x(4:6);
omega_des = r(4:6);
e_omega   = omega - omega_des;

d_roll = sliderconcave(e_omega(1)*2,d_roll);
d_pitch = sliderconcave(e_omega(2)*2,d_pitch);
d_yaw = sliderconcave(e_omega(3)*2,d_yaw);
K_d = diag([d_roll, d_pitch, d_yaw]);

%% Compute controller output
% Apply gains given as parameters
tau = - K_p * e_R_vec - K_d * e_omega;

end

function R = R_euler(Phi)
%R_EULER Function that maps the Z-Y-X Euler angles to the corresponding
%rotation matrix

phi = Phi(1); theta = Phi(2); psi = Phi(3);

R = [  cos(psi)*cos(theta)  cos(psi)*sin(theta)*sin(phi)-sin(psi)*cos(phi)  cos(psi)*cos(phi)*sin(theta)+sin(psi)*sin(phi) ;
       sin(psi)*cos(theta)  sin(psi)*sin(theta)*sin(phi)+cos(psi)*cos(phi)  sin(psi)*cos(phi)*sin(theta)-cos(psi)*sin(phi) ;
      -sin(theta)           cos(theta)*sin(phi)                             cos(theta)*cos(phi)                            ];
end

== matlab function Concave_hipp/concavepd/MATLAB Function1 ==
  data: theta_des input; theta_des output; x input
function theta_des = fcn(theta_des, x)
yaw = x(6);
yaw_des = theta_des(3);
e_yaw = yaw_des-yaw;

% jump from -pi to +pi
if (e_yaw > pi)
    yaw_des = yaw_des - 2*pi;
% jump from +pi to -pi
elseif (-e_yaw > pi)
    yaw_des = yaw_des + 2*pi;
end
theta_des(3) = yaw_des;

== matlab function Concave_hipp/concavepd/Pos controller ==
  data: r input; x input; u output; theta_des output; k_pos input; k_vel input
function [u,theta_des] = fcn(r, x,k_pos,k_vel)
%% Heuristic position controller
% Just wrap around a hueristic position controller around the attitude
% controller
%
% Gains that work for backup
% k_pos=2;
% k_vel=2;
e=r(1:3,1)-x(1:3,1);

k_pos=sliderconcave(e'*e,k_pos);

drive_forward=1; % Easier to drive the unicycle backward than forward
if drive_forward==1
    e=r(1:3,1)-x(1:3,1);
    v_des=k_pos*norm(e,2);
else
    e=x(1:3,1)-r(1:3,1);
    v_des=-k_pos*norm(e,2);    
end

k_vel = sliderconcave(v_des*2,k_vel);
u=k_vel*(v_des-x(4));
proj_dist_xy=norm(e(1:2,1),2);
pitch_des=-atan2(e(3,1),proj_dist_xy);
psi_des=atan2(e(2),e(1));
theta_des=[0;pitch_des;psi_des]; 
end

== matlab function Concave_hipp/concavepd/Subsystem1/MATLAB Function ==
  data: u input; y output
function y = fcn(u)
y = mod(u + pi, 2*pi) - pi;

== matlab function Concave_hipp/HippCampus3/MATLAB Function ==
  data: x input; dx output; in input

function dx = fcn(x, in)
zg    =  0.05;    % [m]
g     =  9.81;    % [m/s^2]

m     =  1.43;    % [kg]
Ix    = 0.00241; % [kgm^2]
Iy    = 0.01072; % [kgm^2]
Iz    = 0.01072; % [kgm^2]
Xudot = -1.11;    % [kg]
Yvdot = -2.80;    % [kg]
Zwdot = -2.80;    % [kg]
Kpdot = -0.0018;  % [kgm^2]
Mqdot = -0.0095;  % [kgm^2]
Nrdot = -0.0095;  % [kgm^2]
Xu    = -4.56;    % [kg/m]
Yv    = -17.36;   % [kg/m]
Zw    = -17.36;   % [kg/m]
Kp    = -0.0028;  % [kgm^2]
Mq    = -0.0476;  % [kgm^2]
Nr    = -0.0476;  % [kgm^2]
% Extract states into more readable form
phi = x( 4); theta = x( 5);
u   = x( 7); v     = x( 8); w   = x( 9);
p   = x(10); q     = x(11); r   = x(12);
nu  = x(7:12);

% Construct rotational tensor
R = body_frame_rotation(x(4:6));

% Construct velocity transformation tensor
T = [ 1  sin(phi)*tan(theta)   cos(phi)*tan(theta) ;
    0  cos(phi)             -sin(phi)            ;
    0  sin(phi)/cos(theta)   cos(phi)/cos(theta) ];
J = [ R         zeros(3) ;
    zeros(3)  T        ];

% Calculate mass matrix
Ma  = -diag([Xudot, Yvdot, Zwdot, Kpdot, Mqdot, Nrdot]);
Mrb =  diag([m,  m,  m, Ix, Iy, Iz]);
M = Ma + Mrb;

% Compute hydrostatic load
gravity = zg * g * m;
G = [ 0; 0; 0; gravity * cos(theta) * sin(phi); gravity * sin(theta); 0 ];

% Construct coriolis matrix, see Fossen 2011, Theorem 3.2
C12 = -skew(M(1:3,1:3) * nu(1:3));
C = [ zeros(3)   C12                        ;
    C12       -skew(M(4:6,4:6) * nu(4:6)) ];

% Construct damping matrix
D = -diag([Xu * abs(u), Yv * abs(v),...
    Zw * abs(w), Kp * abs(p),...
    Mq * abs(q), Nr * abs(r)]);

% Build state space equations
tau  = [ in(1); 0; 0; in(2:4) ];

dx       = zeros(12,1);
dx(1:6)  = J*nu;
dx(7:12) = M \ (tau - (C+D)*nu - G);
end

== matlab function Concave_hipp/HippCampus3/sat1 ==
  data: u input; u_sat output; omega output
function [u_sat, omega] = fcn(u)
  %  u_sat=u;
    h     = 0.0481;   % [m] Distance of rotors to HippoCampus center
    Cd    = 0.0024;   % Coefficient of drag for the rotors
    tlim  = 3;        % Maximal torque of the motors 

    Q = [1,1,1,1;-Cd,Cd,-Cd,Cd;-h,-h,h,h;h,-h,-h,h];
    Qinv = inv(Q);

    % Transform into rotor space
    omega = Qinv*u;

    % Calculate utilization of each rotor
    util  = abs(omega/tlim);

    % Saturate torque at max utilization
    omega = omega ./ max(util, 1);    

    %Transform back into body frame
   u_sat = Q * omega;
end

== matlab function Concave_hipp/MATLAB Function ==
  data: t input; d output
function d = fcn(t)

d = zeros(12,1);

d(7) = 0.2*sin(0.1*t+1);
d(8) = 0.1*sin(0.15*t+0.9);
d(9) = 0.1*sin(0.1*t+0.5);
d(10) = 0.1*sin(0.05*t+1);
d(11) = 0.1*sin(0.1*t+2);
d(12) =0.1*sin(0.15*t+3);

end

== matlab function Concave_hipp/passive error ==
  data: u input; y output
function y = fcn(u)

y = norm(u,2);

== matlab function Concave_hipp/concave passive error ==
  data: u input; y output
function y = fcn(u)

y = norm(u,2);

== matlab function Concave_hipp/concave passive error1 ==
  data: u input; y output
function y = fcn(u)

y = norm(u,2);

== matlab function Concave_hipp/concave passive error2 ==
  data: u input; y output
function y = fcn(u)

y = norm(u,2);

== matlab function Concave_hipp/Passive Controller/Passive Sigma1 ==
  data: ref input; nu_f output; nu_f2 output; s input; Q1 input; Theta_d output; y1m output
%---------------------------------------------------------------------------------------------
% For Paper, 
% "Three-Dimensional Simultaneous Stabilization and Tracking Control of Nonholonomic Autonomous Underwater Vehicles"
% by Shuyuan Fan and Herbert Werner
% Copyright (c) Institute of Control Systems, Hamburg University of Technology. All rights reserved.
% Licensed under the GPLv3. See LICENSE in the project root for license information.
% Uses an own implementation of the work of 
% IEEE Conference on Decision and Control and L-CSS, 2022."
% Author(s): Shuyuan Fan
%--------------------------------------------------------------------------------------------
function [nu_f,nu_f2,Theta_d,y1m]= fcn(ref,s,Q1)
zg    =  0.05;    % [m]
g     =  9.81;    % [m/s^2]

m     =  1.43;    % [kg]
Ix    = 0.00241; % [kgm^2]
Iy    = 0.01072; % [kgm^2]
Iz    = 0.01072; % [kgm^2]
Xudot = -1.11;    % [kg]
Yvdot = -2.80;    % [kg]
Zwdot = -2.80;    % [kg]
Kpdot = -0.0018;  % [kgm^2]
Mqdot = -0.0095;  % [kgm^2]
Nrdot = -0.0095;  % [kgm^2]
Xu    = -4.56;    % [kg/m]
Yv    = -17.36;   % [kg/m]
Zw    = -17.36;   % [kg/m]
Kp    = -0.0028;  % [kgm^2]
Mq    = -0.0476;  % [kgm^2]
Nr    = -0.0476;  % [kgm^2]

% Calculate mass matrix
Ma  = -diag([Xudot, Yvdot, Zwdot, Kpdot, Mqdot, Nrdot]);
Mrb =  diag([m,  m,  m, Ix, Iy, Iz]);
M = Ma + Mrb;

M1 = M(1:3,1:3);
%% reference
x_ref = ref(1);
y_ref = ref(2);
z_ref = ref(3);
Xref = [x_ref;y_ref;z_ref];

%% states
x = s(1); y = s(2); z = s(3);
X = s(1:3);

angle = s(4:6);
phi = s(4);
%phi =min(max(phi,-0.5),0.5);
theta = s(5); 
%theta = min(max(theta,-1.5),1.5);
psi = s(6);
%psi =  wrapToPi(psi);
nu = s(7:9) ;
u=s(7); v=s(8); w=s(9); 

omega = s(10:12);
p=s(10); q=s(11); r=s(12);

% storage function V1
V1 = 0.5*(X-Xref)'*(X-Xref);

% Gamma function for nu
if u<0.5
    nu_u = 0.5;
else
    nu_u = u;
end

nu = [nu_u;v;w];
Gamma_nu = vectortodirect(nu);


% R(Theta)
Rotation = body_frame_rotation(angle);
y1m = Gamma_nu'*Rotation'*(X-Xref);

nu_f = Q1*y1m;
nu_f2 = Gamma_nu*nu_f;

%% Theta_d

Xe = X-Xref;
phi_d  = 0;
theta_d = atan2(Xe(3),sqrt(Xe(1)^2+Xe(2)^2)+eps);
psi_d = atan2(-Xe(2),-Xe(1));
psi_d = wrapTo2Pi(psi_d);
Theta_d = [phi_d;theta_d;psi_d];
end

== matlab function Concave_hipp/Passive Controller/Passive Sigma2 ==
  data: s input; nu_f input; nu_f_dot input; f output; Q2 input
%---------------------------------------------------------------------------------------------
% For Paper, 
% "Three-Dimensional Simultaneous Stabilization and Tracking Control of Nonholonomic Autonomous Underwater Vehicles"
% by Shuyuan Fan and Herbert Werner
% Copyright (c) Institute of Control Systems, Hamburg University of Technology. All rights reserved.
% Licensed under the GPLv3. See LICENSE in the project root for license information.
% Uses an own implementation of the work of 
% IEEE Conference on Decision and Control and L-CSS, 2022."
% Author(s): Shuyuan Fan
%--------------------------------------------------------------------------------------------
function f= fcn(s,nu_f,nu_f_dot,Q2)
zg    =  0.05;    % [m]
g     =  9.81;    % [m/s^2]

m     =  1.43;    % [kg]
Ix    = 0.00241; % [kgm^2]
Iy    = 0.01072; % [kgm^2]
Iz    = 0.01072; % [kgm^2]
Xudot = -1.11;    % [kg]
Yvdot = -2.80;    % [kg]
Zwdot = -2.80;    % [kg]
Kpdot = -0.0018;  % [kgm^2]
Mqdot = -0.0095;  % [kgm^2]
Nrdot = -0.0095;  % [kgm^2]
Xu    = -4.56;    % [kg/m]
Yv    = -17.36;   % [kg/m]
Zw    = -17.36;   % [kg/m]
Kp    = -0.0028;  % [kgm^2]
Mq    = -0.0476;  % [kgm^2]
Nr    = -0.0476;  % [kgm^2]

% Calculate mass matrix
Ma  = -diag([Xudot, Yvdot, Zwdot, Kpdot, Mqdot, Nrdot]);
Mrb =  diag([m,  m,  m, Ix, Iy, Iz]);
M = Ma + Mrb;

M1 = M(1:3,1:3);




%% states
x = s(1); y = s(2); z = s(3);
X = s(1:3);

angle = s(4:6);
phi = s(4);
%phi =min(max(phi,-0.5),0.5);
theta = s(5); 
%theta = min(max(theta,-1.5),1.5);
psi = s(6);
%psi =  wrapToPi(psi);
nu = s(7:9) ;
u=s(7); v=s(8); w=s(9); 

omega = s(10:12);
p=s(10); q=s(11); r=s(12);


% Gamma function for nu
Gamma_nu = vectortodirect(nu);

Gamma_nu_1 = Gamma_nu(1);
if Gamma_nu_1<0.5
    Gamma_nu_1 = 0.5;
end


y2 = u/Gamma_nu_1;
y2star = y2 - nu_f;
% storage function V2
V2 = 0.5*y2star'*Gamma_nu'*M1*M1*Gamma_nu*y2star;


C1 = -skew(M(1:3,1:3) * nu);
D = -diag([Xu * abs(u), Yv * abs(v),...
    Zw * abs(w), Kp * abs(p),...
    Mq * abs(q), Nr * abs(r)]);
D1 = D(1:3,1:3);
H = -C1*omega-D1*nu-M1*nu_f_dot;

Gamma_0 = [1;0;0];
% 
% if abs(Gamma_nu(1))<0.5
%      Gamma_nu(1) = 0.5*sign(Gamma_nu(1));
%  else
%      Gamma_nu(1) = Gamma_nu(1);
%  end

f = (Q2*y2star - H'*M1*Gamma_nu)/((Gamma_0'*M1*Gamma_nu)+eps);
%f = (Q2*y2star - H'*M1*Gamma_nu)/(M1(1,1));
%f=Q2*y2star;


%% Theta_d

end

== matlab function Concave_hipp/HippCampus4/MATLAB Function ==
  data: x input; dx output; in input

function dx = fcn(x, in)
zg    =  0.05;    % [m]
g     =  9.81;    % [m/s^2]

m     =  1.43;    % [kg]
Ix    = 0.00241; % [kgm^2]
Iy    = 0.01072; % [kgm^2]
Iz    = 0.01072; % [kgm^2]
Xudot = -1.11;    % [kg]
Yvdot = -2.80;    % [kg]
Zwdot = -2.80;    % [kg]
Kpdot = -0.0018;  % [kgm^2]
Mqdot = -0.0095;  % [kgm^2]
Nrdot = -0.0095;  % [kgm^2]
Xu    = -4.56;    % [kg/m]
Yv    = -17.36;   % [kg/m]
Zw    = -17.36;   % [kg/m]
Kp    = -0.0028;  % [kgm^2]
Mq    = -0.0476;  % [kgm^2]
Nr    = -0.0476;  % [kgm^2]
% Extract states into more readable form
phi = x( 4); theta = x( 5);
u   = x( 7); v     = x( 8); w   = x( 9);
p   = x(10); q     = x(11); r   = x(12);
nu  = x(7:12);

% Construct rotational tensor
R = body_frame_rotation(x(4:6));

% Construct velocity transformation tensor
T = [ 1  sin(phi)*tan(theta)   cos(phi)*tan(theta) ;
    0  cos(phi)             -sin(phi)            ;
    0  sin(phi)/cos(theta)   cos(phi)/cos(theta) ];
J = [ R         zeros(3) ;
    zeros(3)  T        ];

% Calculate mass matrix
Ma  = -diag([Xudot, Yvdot, Zwdot, Kpdot, Mqdot, Nrdot]);
Mrb =  diag([m,  m,  m, Ix, Iy, Iz]);
M = Ma + Mrb;

% Compute hydrostatic load
gravity = zg * g * m;
G = [ 0; 0; 0; gravity * cos(theta) * sin(phi); gravity * sin(theta); 0 ];

% Construct coriolis matrix, see Fossen 2011, Theorem 3.2
C12 = -skew(M(1:3,1:3) * nu(1:3));
C = [ zeros(3)   C12                        ;
    C12       -skew(M(4:6,4:6) * nu(4:6)) ];

% Construct damping matrix
D = -diag([Xu * abs(u), Yv * abs(v),...
    Zw * abs(w), Kp * abs(p),...
    Mq * abs(q), Nr * abs(r)]);

% Build state space equations
tau  = [ in(1); 0; 0; in(2:4) ];

dx       = zeros(12,1);
dx(1:6)  = J*nu;
dx(7:12) = M \ (tau - (C+D)*nu - G);
end

== matlab function Concave_hipp/Passive Controller/Passive Sigma3 ==
  data: s input; Theta_d input; Theta_d_dot input; omega_f output; Q3 input
%---------------------------------------------------------------------------------------------
% For Paper, 
% "Three-Dimensional Simultaneous Stabilization and Tracking Control of Nonholonomic Autonomous Underwater Vehicles"
% by Shuyuan Fan and Herbert Werner
% Copyright (c) Institute of Control Systems, Hamburg University of Technology. All rights reserved.
% Licensed under the GPLv3. See LICENSE in the project root for license information.
% Uses an own implementation of the work of 
% IEEE Conference on Decision and Control and L-CSS, 2022."
% Author(s): Shuyuan Fan
%--------------------------------------------------------------------------------------------
function omega_f= fcn(s,Theta_d,Theta_d_dot,Q3)

%% states
x = s(1); y = s(2); z = s(3);
X = s(1:3);

%angle = s(4:6);
phi = s(4);
%phi =min(max(phi,-0.5),0.5);
theta = s(5); 
theta = min(max(theta,-1.0),1.0);
psi = s(6);
angle = [phi;theta;psi];
%psi =  wrapToPi(psi);
nu = s(7:9) ;
u=s(7); v=s(8); w=s(9); 

omega = s(10:12);
p=s(10); q=s(11); r=s(12);

phi_d = Theta_d(1);
theta_d = Theta_d(2);
psi_d = Theta_d(3);
%psi_d = atan2(sin(psi_d),cos(psi_d));

% storage function V3
V3 = 0.5*(angle-Theta_d)'*(angle-Theta_d);


T = Jaco(angle);
Q3 = diag(Q3);
y3star = angle-Theta_d;
y3star(3) = atan2(sin(y3star(3)),cos(y3star(3))); 
omega_f = inv(T)*(Q3*y3star+Theta_d_dot);
%omega_f = inv(T)*(Q3*y3star);


end

== matlab function Concave_hipp/Passive Controller/Passive Sigma4 ==
  data: s input; omega_f input; omega_f_dot input; tau2 output; Q4 input
%---------------------------------------------------------------------------------------------
% For Paper, 
% "Three-Dimensional Simultaneous Stabilization and Tracking Control of Nonholonomic Autonomous Underwater Vehicles"
% by Shuyuan Fan and Herbert Werner
% Copyright (c) Institute of Control Systems, Hamburg University of Technology. All rights reserved.
% Licensed under the GPLv3. See LICENSE in the project root for license information.
% Uses an own implementation of the work of 
% IEEE Conference on Decision and Control and L-CSS, 2022."
% Author(s): Shuyuan Fan
%--------------------------------------------------------------------------------------------
function tau2= fcn(s,omega_f,omega_f_dot,Q4)
zg    =  0.05;    % [m]
g     =  9.81;    % [m/s^2]

m     =  1.43;    % [kg]
Ix    = 0.00241; % [kgm^2]
Iy    = 0.01072; % [kgm^2]
Iz    = 0.01072; % [kgm^2]
Xudot = -1.11;    % [kg]
Yvdot = -2.80;    % [kg]
Zwdot = -2.80;    % [kg]
Kpdot = -0.0018;  % [kgm^2]
Mqdot = -0.0095;  % [kgm^2]
Nrdot = -0.0095;  % [kgm^2]
Xu    = -4.56;    % [kg/m]
Yv    = -17.36;   % [kg/m]
Zw    = -17.36;   % [kg/m]
Kp    = -0.0028;  % [kgm^2]
Mq    = -0.0476;  % [kgm^2]
Nr    = -0.0476;  % [kgm^2]

% Calculate mass matrix
Ma  = -diag([Xudot, Yvdot, Zwdot, Kpdot, Mqdot, Nrdot]);
Mrb =  diag([m,  m,  m, Ix, Iy, Iz]);
M = Ma + Mrb;

M1 = M(1:3,1:3);
M2 = M(4:6,4:6);



%% states
x = s(1); y = s(2); z = s(3);
X = s(1:3);

angle = s(4:6);
phi = s(4);
%phi =min(max(phi,-0.5),0.5);
theta = s(5); 
%theta = min(max(theta,-1.5),1.5);
psi = s(6);
%psi =  wrapToPi(psi);
nu = s(7:9) ;
u=s(7); v=s(8); w=s(9); 

omega = s(10:12);
p=s(10); q=s(11); r=s(12);


% Gamma function for nu
Gamma_nu = vectortodirect(nu);

y4 = omega;
y4star = y4 - omega_f;
% storage function V2
%V2 = 0.5*y4star'*Gamma_nu'*M1*M1*Gamma_nu*y4star;


C1 = -skew(M(1:3,1:3) * nu);
C2 = -skew(M(4:6,4:6) * omega);
D = -diag([Xu * abs(u), Yv * abs(v),...
    Zw * abs(w), Kp * abs(p),...
    Mq * abs(q), Nr * abs(r)]);
D1 = D(1:3,1:3);
D2 = D(4:6,4:6);
gravity = zg * g * m;
G = [ 0; 0; 0; gravity * cos(theta) * sin(phi); gravity * sin(theta); 0 ];
g2 = G(4:6);
O = -C1*nu-C2*omega-D2*omega-g2;
Q4 = diag(Q4);
tau2 = inv(M2)*(Q4*y4star-M2*O+M2*M2*omega_f_dot);
%tau2 = inv(M2)*(Q4*y4star-M2*O);

end

== matlab function Concave_hipp/concave Passive Controller1/Passive Sigma2 ==
  data: s input; nu_f input; nu_f_dot input; f output; Q2 input; V2 output
%---------------------------------------------------------------------------------------------
% For Paper, 
% "Three-Dimensional Simultaneous Stabilization and Tracking Control of Nonholonomic Autonomous Underwater Vehicles"
% by Shuyuan Fan and Herbert Werner
% Copyright (c) Institute of Control Systems, Hamburg University of Technology. All rights reserved.
% Licensed under the GPLv3. See LICENSE in the project root for license information.
% Uses an own implementation of the work of 
% IEEE Conference on Decision and Control and L-CSS, 2022."
% Author(s): Shuyuan Fan
%--------------------------------------------------------------------------------------------
function [f,V2]= fcn(s,nu_f,nu_f_dot,Q2)
zg    =  0.05;    % [m]
g     =  9.81;    % [m/s^2]

m     =  1.43;    % [kg]
Ix    = 0.00241; % [kgm^2]
Iy    = 0.01072; % [kgm^2]
Iz    = 0.01072; % [kgm^2]
Xudot = -1.11;    % [kg]
Yvdot = -2.80;    % [kg]
Zwdot = -2.80;    % [kg]
Kpdot = -0.0018;  % [kgm^2]
Mqdot = -0.0095;  % [kgm^2]
Nrdot = -0.0095;  % [kgm^2]
Xu    = -4.56;    % [kg/m]
Yv    = -17.36;   % [kg/m]
Zw    = -17.36;   % [kg/m]
Kp    = -0.0028;  % [kgm^2]
Mq    = -0.0476;  % [kgm^2]
Nr    = -0.0476;  % [kgm^2]

% Calculate mass matrix
Ma  = -diag([Xudot, Yvdot, Zwdot, Kpdot, Mqdot, Nrdot]);
Mrb =  diag([m,  m,  m, Ix, Iy, Iz]);
M = Ma + Mrb;

M1 = M(1:3,1:3);




%% states
x = s(1); y = s(2); z = s(3);
X = s(1:3);

angle = s(4:6);
phi = s(4);
%phi =min(max(phi,-0.5),0.5);
theta = s(5); 
%theta = min(max(theta,-1.5),1.5);
psi = s(6);
%psi =  wrapToPi(psi);
nu = s(7:9) ;
u=s(7); v=s(8); w=s(9); 

omega = s(10:12);
p=s(10); q=s(11); r=s(12);


% Gamma function for nu
Gamma_nu = vectortodirect(nu);

Gamma_nu_1 = Gamma_nu(1);
if Gamma_nu_1<0.5
    Gamma_nu_1 = 0.5;
end


y2 = u/Gamma_nu_1;
y2star = y2 - nu_f;
% storage function V2
V2 = 0.5*y2star'*Gamma_nu'*M1*M1*Gamma_nu*y2star;


C1 = -skew(M(1:3,1:3) * nu);
D = -diag([Xu * abs(u), Yv * abs(v),...
    Zw * abs(w), Kp * abs(p),...
    Mq * abs(q), Nr * abs(r)]);
D1 = D(1:3,1:3);
H = -C1*omega-D1*nu-M1*nu_f_dot;

Gamma_0 = [1;0;0];
% 
% if abs(Gamma_nu(1))<0.5
%      Gamma_nu(1) = 0.5*sign(Gamma_nu(1));
%  else
%      Gamma_nu(1) = Gamma_nu(1);
%  end

Q2 = -sliderconcave(V2,-Q2);

f = (Q2*y2star - H'*M1*Gamma_nu)/((Gamma_0'*M1*Gamma_nu)+eps);
%f = (Q2*y2star - H'*M1*Gamma_nu)/(M1(1,1));
%f=Q2*y2star;


%% Theta_d

end

== matlab function Concave_hipp/concave Passive Controller1/Passive Sigma3 ==
  data: s input; Theta_d input; Theta_d_dot input; omega_f output; Q3 input; V3 output
%---------------------------------------------------------------------------------------------
% For Paper, 
% "Three-Dimensional Simultaneous Stabilization and Tracking Control of Nonholonomic Autonomous Underwater Vehicles"
% by Shuyuan Fan and Herbert Werner
% Copyright (c) Institute of Control Systems, Hamburg University of Technology. All rights reserved.
% Licensed under the GPLv3. See LICENSE in the project root for license information.
% Uses an own implementation of the work of 
% IEEE Conference on Decision and Control and L-CSS, 2022."
% Author(s): Shuyuan Fan
%--------------------------------------------------------------------------------------------
function [omega_f,V3]= fcn(s,Theta_d,Theta_d_dot,Q3)

%% states
x = s(1); y = s(2); z = s(3);
X = s(1:3);

%angle = s(4:6);
phi = s(4);
%phi =min(max(phi,-0.5),0.5);
theta = s(5); 
theta = min(max(theta,-1.0),1.0);
psi = s(6);
angle = [phi;theta;psi];
%psi =  wrapToPi(psi);
nu = s(7:9) ;
u=s(7); v=s(8); w=s(9); 

omega = s(10:12);
p=s(10); q=s(11); r=s(12);

phi_d = Theta_d(1);
theta_d = Theta_d(2);
psi_d = Theta_d(3);
%psi_d = atan2(sin(psi_d),cos(psi_d));

% storage function V3
V3 = 0.5*(angle-Theta_d)'*(angle-Theta_d);


q31 = -sliderconcave(V3,-Q3(1,:));
q32 = -sliderconcave(V3,-Q3(2,:));
q33 = -sliderconcave(V3,-Q3(3,:));
Q3 = diag([q31,q32,q33]);
T = Jaco(angle);

y3star = angle-Theta_d;
y3star(3) = atan2(sin(y3star(3)),cos(y3star(3))); 
omega_f = inv(T)*(Q3*y3star+Theta_d_dot);
%omega_f = inv(T)*(Q3*y3star);


end

== matlab function Concave_hipp/concave Passive Controller1/Passive Sigma4 ==
  data: s input; omega_f input; omega_f_dot input; tau2 output; Q4 input; V4 output
%---------------------------------------------------------------------------------------------
% For Paper, 
% "Three-Dimensional Simultaneous Stabilization and Tracking Control of Nonholonomic Autonomous Underwater Vehicles"
% by Shuyuan Fan and Herbert Werner
% Copyright (c) Institute of Control Systems, Hamburg University of Technology. All rights reserved.
% Licensed under the GPLv3. See LICENSE in the project root for license information.
% Uses an own implementation of the work of 
% IEEE Conference on Decision and Control and L-CSS, 2022."
% Author(s): Shuyuan Fan
%--------------------------------------------------------------------------------------------
function [tau2,V4]= fcn(s,omega_f,omega_f_dot,Q4)
zg    =  0.05;    % [m]
g     =  9.81;    % [m/s^2]

m     =  1.43;    % [kg]
Ix    = 0.00241; % [kgm^2]
Iy    = 0.01072; % [kgm^2]
Iz    = 0.01072; % [kgm^2]
Xudot = -1.11;    % [kg]
Yvdot = -2.80;    % [kg]
Zwdot = -2.80;    % [kg]
Kpdot = -0.0018;  % [kgm^2]
Mqdot = -0.0095;  % [kgm^2]
Nrdot = -0.0095;  % [kgm^2]
Xu    = -4.56;    % [kg/m]
Yv    = -17.36;   % [kg/m]
Zw    = -17.36;   % [kg/m]
Kp    = -0.0028;  % [kgm^2]
Mq    = -0.0476;  % [kgm^2]
Nr    = -0.0476;  % [kgm^2]

% Calculate mass matrix
Ma  = -diag([Xudot, Yvdot, Zwdot, Kpdot, Mqdot, Nrdot]);
Mrb =  diag([m,  m,  m, Ix, Iy, Iz]);
M = Ma + Mrb;

M1 = M(1:3,1:3);
M2 = M(4:6,4:6);



%% states
x = s(1); y = s(2); z = s(3);
X = s(1:3);

angle = s(4:6);
phi = s(4);
%phi =min(max(phi,-0.5),0.5);
theta = s(5); 
%theta = min(max(theta,-1.5),1.5);
psi = s(6);
%psi =  wrapToPi(psi);
nu = s(7:9) ;
u=s(7); v=s(8); w=s(9); 

omega = s(10:12);
p=s(10); q=s(11); r=s(12);


% Gamma function for nu
Gamma_nu = vectortodirect(nu);

y4 = omega;
y4star = y4 - omega_f;
% storage function V2
V4 = 0.5*y4star'*M2*M2*y4star;

q41 = -sliderconcave(V4,-Q4(1,:));
q42 = -sliderconcave(V4,-Q4(2,:));
q43 = -sliderconcave(V4,-Q4(3,:));
Q4 = diag([q41,q42,q43]);

C1 = -skew(M(1:3,1:3) * nu);
C2 = -skew(M(4:6,4:6) * omega);
D = -diag([Xu * abs(u), Yv * abs(v),...
    Zw * abs(w), Kp * abs(p),...
    Mq * abs(q), Nr * abs(r)]);
D1 = D(1:3,1:3);
D2 = D(4:6,4:6);
gravity = zg * g * m;
G = [ 0; 0; 0; gravity * cos(theta) * sin(phi); gravity * sin(theta); 0 ];
g2 = G(4:6);
O = -C1*nu-C2*omega-D2*omega-g2;
tau2 = inv(M2)*(Q4*y4star-M2*O+M2*M2*omega_f_dot);
%tau2 = inv(M2)*(Q4*y4star-M2*O);

end

== matlab function Concave_hipp/HippCampus1/MATLAB Function ==
  data: x input; dx output; in input

function dx = fcn(x, in)
zg    =  0.05;    % [m]
g     =  9.81;    % [m/s^2]

m     =  1.43;    % [kg]
Ix    = 0.00241; % [kgm^2]
Iy    = 0.01072; % [kgm^2]
Iz    = 0.01072; % [kgm^2]
Xudot = -1.11;    % [kg]
Yvdot = -2.80;    % [kg]
Zwdot = -2.80;    % [kg]
Kpdot = -0.0018;  % [kgm^2]
Mqdot = -0.0095;  % [kgm^2]
Nrdot = -0.0095;  % [kgm^2]
Xu    = -4.56;    % [kg/m]
Yv    = -17.36;   % [kg/m]
Zw    = -17.36;   % [kg/m]
Kp    = -0.0028;  % [kgm^2]
Mq    = -0.0476;  % [kgm^2]
Nr    = -0.0476;  % [kgm^2]
% Extract states into more readable form
phi = x( 4); theta = x( 5);
u   = x( 7); v     = x( 8); w   = x( 9);
p   = x(10); q     = x(11); r   = x(12);
nu  = x(7:12);

% Construct rotational tensor
R = body_frame_rotation(x(4:6));

% Construct velocity transformation tensor
T = [ 1  sin(phi)*tan(theta)   cos(phi)*tan(theta) ;
    0  cos(phi)             -sin(phi)            ;
    0  sin(phi)/cos(theta)   cos(phi)/cos(theta) ];
J = [ R         zeros(3) ;
    zeros(3)  T        ];

% Calculate mass matrix
Ma  = -diag([Xudot, Yvdot, Zwdot, Kpdot, Mqdot, Nrdot]);
Mrb =  diag([m,  m,  m, Ix, Iy, Iz]);
M = Ma + Mrb;

% Compute hydrostatic load
gravity = zg * g * m;
G = [ 0; 0; 0; gravity * cos(theta) * sin(phi); gravity * sin(theta); 0 ];

% Construct coriolis matrix, see Fossen 2011, Theorem 3.2
C12 = -skew(M(1:3,1:3) * nu(1:3));
C = [ zeros(3)   C12                        ;
    C12       -skew(M(4:6,4:6) * nu(4:6)) ];

% Construct damping matrix
D = -diag([Xu * abs(u), Yv * abs(v),...
    Zw * abs(w), Kp * abs(p),...
    Mq * abs(q), Nr * abs(r)]);

% Build state space equations
tau  = [ in(1); 0; 0; in(2:4) ];

dx       = zeros(12,1);
dx(1:6)  = J*nu;
dx(7:12) = M \ (tau - (C+D)*nu - G);
end

== matlab function Concave_hipp/HippCampus1/sat1 ==
  data: u input; u_sat output; omega output
function [u_sat, omega] = fcn(u)
  %  u_sat=u;
    h     = 0.0481;   % [m] Distance of rotors to HippoCampus center
    Cd    = 0.0024;   % Coefficient of drag for the rotors
    tlim  = 3;        % Maximal torque of the motors 

    Q = [1,1,1,1;-Cd,Cd,-Cd,Cd;-h,-h,h,h;h,-h,-h,h];
    Qinv = inv(Q);

    % Transform into rotor space
    omega = Qinv*u;

    % Calculate utilization of each rotor
    util  = abs(omega/tlim);

    % Saturate torque at max utilization
    omega = omega ./ max(util, 1);    

    %Transform back into body frame
   u_sat = Q * omega;
end
